simulink model "pendulum"  (R2022b)
settings: Solver=VariableStepAuto  StartTime=0.0  StopTime=10.0  RelTol=1e-3
settings Model: Creator=henry  LastModifiedBy=henry

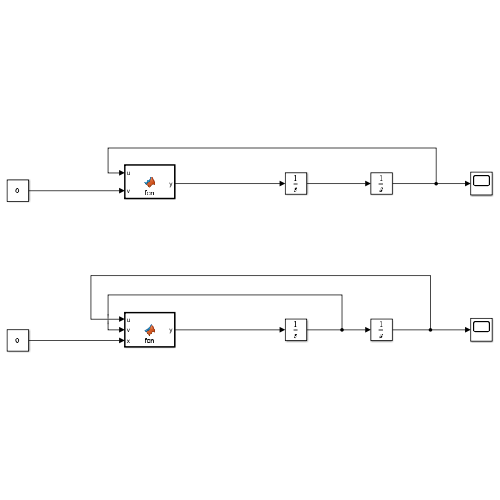
[thumbnail: Simulink's stored preview of the top-level diagram]
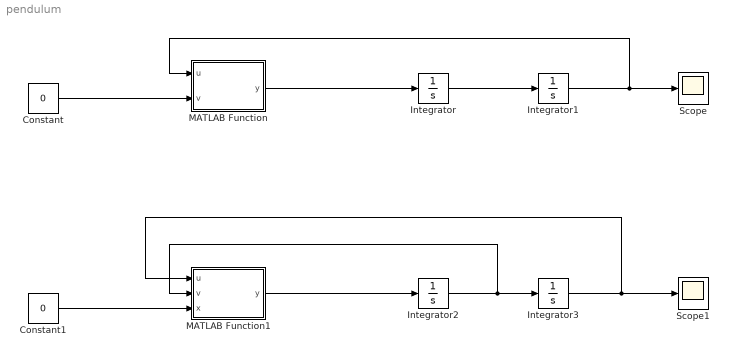
== system pendulum ==
  Constant : Constant  Value=0
  Constant1 : Constant  Value=0
  Integrator : Integrator  InitialCondition=30*pi/180
  Integrator1 : Integrator
  Integrator2 : Integrator  InitialCondition=30*pi/180
  Integrator3 : Integrator
  MATLAB Function : MATLAB Function  TreatAsAtomicUnit=on
  MATLAB Function1 : MATLAB Function  TreatAsAtomicUnit=on
  Scope : Scope
  Scope1 : Scope
  wires:
  Constant/1 -> MATLAB Function/2(v)
  MATLAB Function/1(y) -> Integrator/1
  Integrator/1 -> Integrator1/1
  Integrator1/1 -> MATLAB Function/1(u), Scope/1
  MATLAB Function1/1(y) -> Integrator2/1
  Integrator2/1 -> MATLAB Function1/2(v), Integrator3/1
  Integrator3/1 -> MATLAB Function1/1(u), Scope1/1
  Constant1/1 -> MATLAB Function1/3(x)

== matlab function pendulum/MATLAB Function ==
  data: u input; y output; v input
function y = fcn(u, v)

y = -9.81/1.0*sin(u) + 1/0.05/1.0^2*v;

== matlab function pendulum/MATLAB Function1 ==
  data: u input; y output; v input; x input
function y = fcn(u, v, x)

y = -9.81/1.0*sin(u) - 0.05/0.05/1.0*v + 1/0.05/1.0^2*x;
